simulink model "SpinningMode"  (R2024b)
settings: Solver=FixedStepAuto  StartTime=0.0  StopTime=10.0  RelTol=1e-3  EnableMultiTasking=on
undefined symbols (not defined in the file): MSpin, nRPMSpinningModeIntegralActivation, NSpinningModeKi, NSpinningModelKp, nTargetRPM, tSpinLength, tTorqueControlTask
libraries: simulink x3, simulink_extras x1
settings Model: DataDictionary=Master_Dictionary.sldd  EnableAccessToBaseWorkspace=off  Creator=torni  LastModifiedBy=Will
settings OptimizationCC: DefaultParameterBehavior=Inlined  EnhancedBackFolding=on  PassReuseOutputArgsAs=Individual arguments  ZeroExternalMemoryAtStartup=off  ZeroInternalMemoryAtStartup=off  MaxStackSize=8192  OptimizeBlockOrder=speed  DifferentSizesBufferReuse=on  OptimizationCustomize=off  EfficientTunableParamExpr=on
settings DebuggingCC: ParameterTunabilityLossMsg=error
settings HardwareCC: ProdBitPerPointer=32  ProdBitPerSizeT=32  ProdBitPerPtrDiffT=32  ProdLargestAtomicInteger=Long  ProdLargestAtomicFloat=Double  ProdWordSize=32  ProdLongLongMode=on  ProdHWDeviceType=ARM Compatible->ARM Cortex-M
settings SFSimCC: MATLABDynamicMemAlloc=off
settings RTWCC: Description=Embedded Coder  SystemTargetFile=ert.tlc  HardwareBoard=STM32H7xx Based (Single-core)  TemplateMakefile=ert_default_tmf  Toolchain=GNU Tools for ARM Embedded Processors
settings CodeAppCC: ForceParamTrailComments=on  IgnoreCustomStorageClasses=off  OperatorAnnotations=on  SimulinkDataObjDesc=on  SFDataObjDesc=on  InsertBlockDesc=on
settings ERTTargetCC: TargetLangStandard=C99 (ISO)  CodeReplacementLibrary=ARM Cortex-M  ExtModeTransport=3  ExtModeStaticAlloc=on  ExtModeStaticAllocSize=2048  ExtModeMexFile=ext_xcp  ExtModeIntrfLevel=Level2 - Open

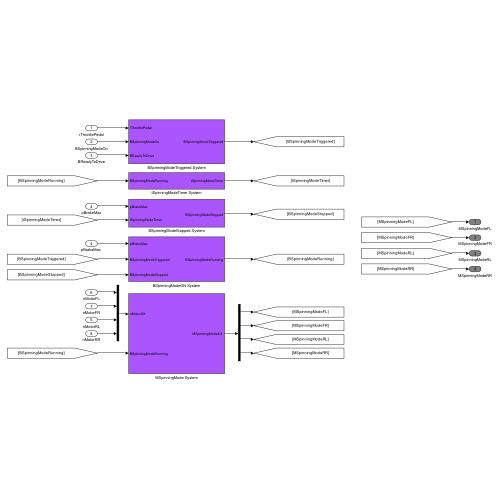
[thumbnail: Simulink's stored preview of the top-level diagram]
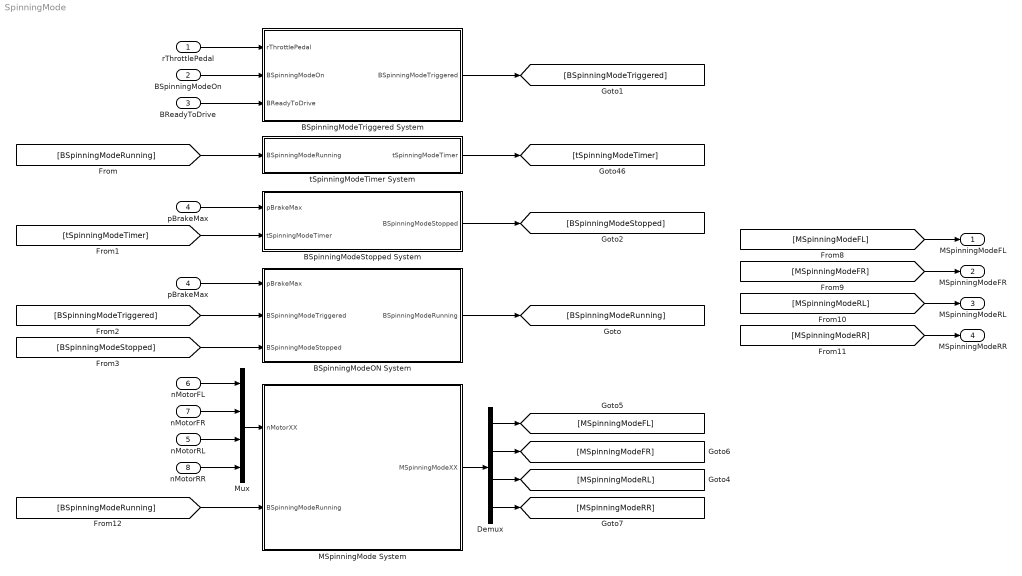
== system SpinningMode ==
  rThrottlePedal : Inport  OutDataTypeStr=double
  "BSpinningModeOn " : Inport  Port=2  OutDataTypeStr=boolean
  BReadyToDrive : Inport  Port=3  OutDataTypeStr=boolean
  pBrakeMax : Inport  Port=4  OutDataTypeStr=double
  nMotorRL : Inport  Port=5  OutDataTypeStr=double
  nMotorFL : Inport  Port=6  OutDataTypeStr=double
  nMotorFR : Inport  Port=7  OutDataTypeStr=double
  nMotorRR : Inport  Port=8  OutDataTypeStr=double
  BSpinningModeON System : Subsystem
  BSpinningModeStopped System : Subsystem
  BSpinningModeTriggered System : Subsystem
  Demux : Demux
  MSpinningMode System : Subsystem
  Mux : Mux
  "pBrakeMax " : InportShadow  Port=4  OutDataTypeStr=double
  tSpinningModeTimer System : Subsystem
  MSpinningModeFL : Outport  OutDataTypeStr=double  VectorParamsAs1DForOutWhenUnconnected=off
  MSpinningModeFR : Outport  Port=2  OutDataTypeStr=double  VectorParamsAs1DForOutWhenUnconnected=off
  MSpinningModeRL : Outport  Port=3  OutDataTypeStr=double  VectorParamsAs1DForOutWhenUnconnected=off
  MSpinningModeRR : Outport  Port=4  OutDataTypeStr=double  VectorParamsAs1DForOutWhenUnconnected=off
  wires:
  rThrottlePedal/1 -> BSpinningModeTriggered System/1(rThrottlePedal)
  "BSpinningModeOn "/1 -> BSpinningModeTriggered System/2("BSpinningModeOn ")
  BReadyToDrive/1 -> BSpinningModeTriggered System/3(BReadyToDrive)
  pBrakeMax/1 -> BSpinningModeStopped System/1(pBrakeMax)
  [tSpinningModeTimer] -> BSpinningModeStopped System/2(tSpinningModeTimer)
  tSpinningModeTimer System/1(tSpinningModeTimer) -> [tSpinningModeTimer]
  BSpinningModeTriggered System/1(BSpinningModeTriggered) -> [BSpinningModeTriggered]
  BSpinningModeStopped System/1(BSpinningModeStopped) -> [BSpinningModeStopped]
  "pBrakeMax "/1 -> BSpinningModeON System/1(pBrakeMax)
  [BSpinningModeTriggered] -> BSpinningModeON System/2(BSpinningModeTriggered)
  [BSpinningModeStopped] -> BSpinningModeON System/3(BSpinningModeStopped)
  BSpinningModeON System/1(BSpinningModeRunning) -> [BSpinningModeRunning]
  [BSpinningModeRunning] -> tSpinningModeTimer System/1(BSpinningModeRunning)
  Demux/3 -> [MSpinningModeRL]
  Demux/1 -> [MSpinningModeFL]
  Demux/2 -> [MSpinningModeFR]
  Demux/4 -> [MSpinningModeRR]
  [MSpinningModeFL] -> MSpinningModeFL/1
  [MSpinningModeFR] -> MSpinningModeFR/1
  [MSpinningModeRR] -> MSpinningModeRR/1
  [MSpinningModeRL] -> MSpinningModeRL/1
  Mux/1 -> MSpinningMode System/1(nMotorXX)
  nMotorFL/1 -> Mux/1
  nMotorFR/1 -> Mux/2
  nMotorRL/1 -> Mux/3
  nMotorRR/1 -> Mux/4
  [BSpinningModeRunning] -> MSpinningMode System/2(BSpinningModeRunning)
  MSpinningMode System/1("MSpinningModeXX ") -> Demux/1

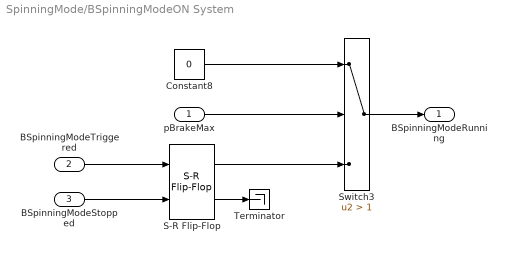
== system SpinningMode/BSpinningModeON System ==
  pBrakeMax : Inport  OutDataTypeStr=double
  BSpinningModeTriggered : Inport  Port=2  OutDataTypeStr=boolean
  BSpinningModeStopped : Inport  Port=3  OutDataTypeStr=boolean
  Constant8 : Constant  Value=0
  S-R Flip-Flop : simulink_extras/Flip Flops/S-R Flip-Flop  initial_condition=0
  Switch3 : Switch  Criteria=u2 > Threshold  Threshold=1  SaturateOnIntegerOverflow=off  InputSameDT=off
  Terminator : Terminator
  BSpinningModeRunning : Outport  OutDataTypeStr=boolean  VectorParamsAs1DForOutWhenUnconnected=off
  wires:
  Switch3/1 -> BSpinningModeRunning/1
  BSpinningModeTriggered/1 -> S-R Flip-Flop/1
  Constant8/1 -> Switch3/1
  S-R Flip-Flop/1 -> Switch3/3
  S-R Flip-Flop/2 -> Terminator/1
  BSpinningModeStopped/1 -> S-R Flip-Flop/2
  pBrakeMax/1 -> Switch3/2

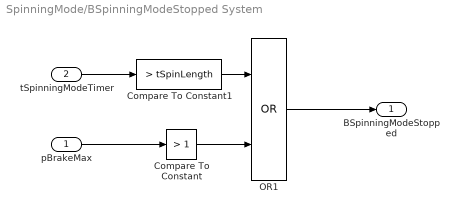
== system SpinningMode/BSpinningModeStopped System ==
  pBrakeMax : Inport  OutDataTypeStr=double
  tSpinningModeTimer : Inport  Port=2  OutDataTypeStr=double
  Compare To Constant : simulink/Logic and Bit Operations/Compare To Constant  relop=>  const=1  OutDataTypeStr=boolean
  Compare To Constant1 : simulink/Logic and Bit Operations/Compare To Constant  relop=>  const=tSpinLength  OutDataTypeStr=boolean
  OR1 : Logic  Operator=OR  AllPortsSameDT=off  OutDataTypeStr=boolean
  BSpinningModeStopped : Outport  OutDataTypeStr=boolean  VectorParamsAs1DForOutWhenUnconnected=off
  wires:
  Compare To Constant1/1 -> OR1/1
  Compare To Constant/1 -> OR1/2
  OR1/1 -> BSpinningModeStopped/1
  pBrakeMax/1 -> Compare To Constant/1
  tSpinningModeTimer/1 -> Compare To Constant1/1

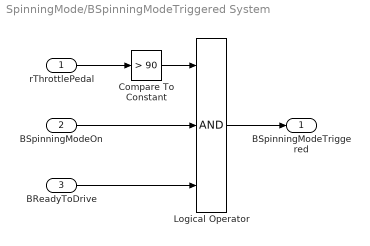
== system SpinningMode/BSpinningModeTriggered System ==
  rThrottlePedal : Inport  OutDataTypeStr=double
  "BSpinningModeOn " : Inport  Port=2  OutDataTypeStr=boolean
  BReadyToDrive : Inport  Port=3  OutDataTypeStr=boolean
  Compare To Constant : simulink/Logic and Bit Operations/Compare To Constant  relop=>  const=90  OutDataTypeStr=boolean
  Logical Operator : Logic  Inputs=3  AllPortsSameDT=off  OutDataTypeStr=boolean
  BSpinningModeTriggered : Outport  OutDataTypeStr=boolean  VectorParamsAs1DForOutWhenUnconnected=off
  wires:
  Logical Operator/1 -> BSpinningModeTriggered/1
  "BSpinningModeOn "/1 -> Logical Operator/2
  rThrottlePedal/1 -> Compare To Constant/1
  Compare To Constant/1 -> Logical Operator/1
  BReadyToDrive/1 -> Logical Operator/3

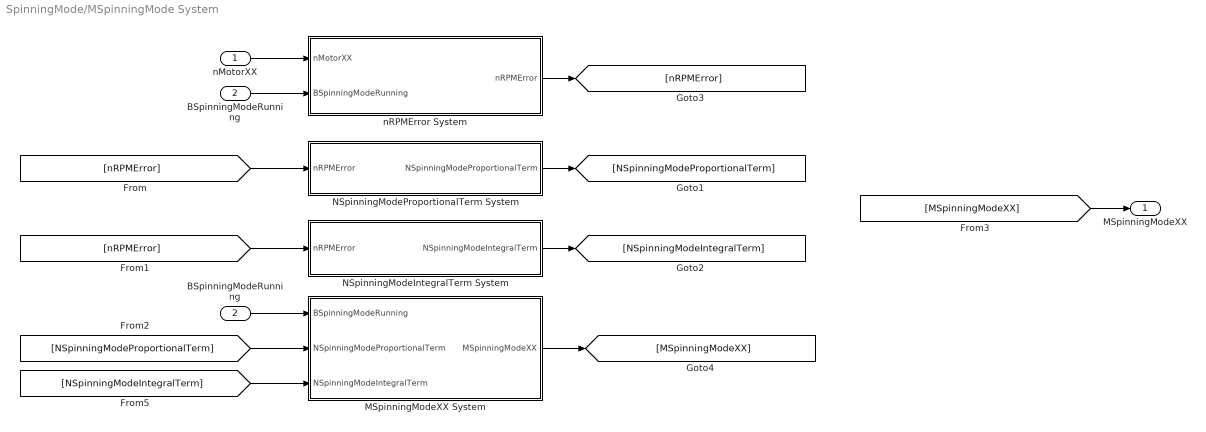
== system SpinningMode/MSpinningMode System ==
  nMotorXX : Inport  OutDataTypeStr=double
  BSpinningModeRunning : Inport  Port=2  OutDataTypeStr=boolean
  "BSpinningModeRunning " : InportShadow  Port=2  OutDataTypeStr=boolean
  MSpinningModeXX System : Subsystem
  NSpinningModeIntegralTerm System : Subsystem
  NSpinningModeProportionalTerm System : Subsystem
  nRPMError System : Subsystem
  "MSpinningModeXX " : Outport  OutDataTypeStr=double  VectorParamsAs1DForOutWhenUnconnected=off
  wires:
  nMotorXX/1 -> nRPMError System/1(nMotorXX)
  BSpinningModeRunning/1 -> nRPMError System/2(BSpinningModeRunning)
  nRPMError System/1(nRPMError) -> [nRPMError]
  [nRPMError] -> NSpinningModeProportionalTerm System/1(nRPMError)
  NSpinningModeProportionalTerm System/1(NSpinningModeProportionalTerm) -> [NSpinningModeProportionalTerm]
  [nRPMError] -> NSpinningModeIntegralTerm System/1(nRPMError)
  NSpinningModeIntegralTerm System/1("NSpinningModeIntegralTerm ") -> [NSpinningModeIntegralTerm]
  [NSpinningModeProportionalTerm] -> MSpinningModeXX System/2(NSpinningModeProportionalTerm)
  [NSpinningModeIntegralTerm] -> MSpinningModeXX System/3(NSpinningModeIntegralTerm)
  "BSpinningModeRunning "/1 -> MSpinningModeXX System/1(BSpinningModeRunning)
  MSpinningModeXX System/1("MSpinningModeXX ") -> [MSpinningModeXX]
  [MSpinningModeXX] -> "MSpinningModeXX "/1

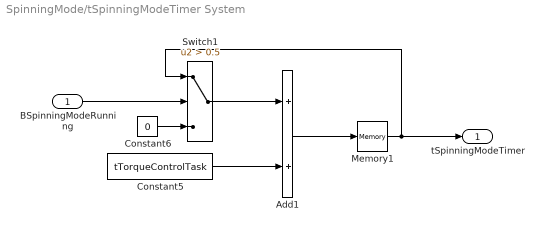
== system SpinningMode/tSpinningModeTimer System ==
  BSpinningModeRunning : Inport  OutDataTypeStr=boolean
  Add1 : Sum
  Constant5 : Constant  Value=tTorqueControlTask
  Constant6 : Constant  Value=0
  Memory1 : Memory  InheritSampleTime=on
  Switch1 : Switch  Criteria=u2 > Threshold  Threshold=0.5  SaturateOnIntegerOverflow=off  InputSameDT=off
  tSpinningModeTimer : Outport  OutDataTypeStr=double  VectorParamsAs1DForOutWhenUnconnected=off
  wires:
  Add1/1 -> Memory1/1
  Memory1/1 -> tSpinningModeTimer/1, Switch1/1
  Switch1/1 -> Add1/1
  Constant5/1 -> Add1/2
  Constant6/1 -> Switch1/3
  BSpinningModeRunning/1 -> Switch1/2

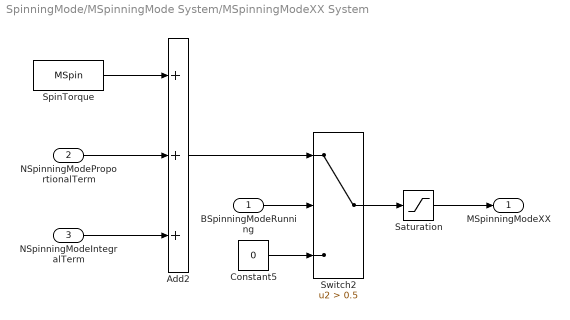
== system SpinningMode/MSpinningMode System/MSpinningModeXX System ==
  BSpinningModeRunning : Inport  OutDataTypeStr=boolean
  NSpinningModeProportionalTerm : Inport  Port=2  OutDataTypeStr=double
  NSpinningModeIntegralTerm : Inport  Port=3  OutDataTypeStr=double
  Add2 : Sum  Inputs=+++
  Constant5 : Constant  Value=0
  Saturation : Saturate  UpperLimit=15  LowerLimit=0
  SpinTorque : Constant  Value=MSpin
  Switch2 : Switch  Criteria=u2 > Threshold  Threshold=0.5  SaturateOnIntegerOverflow=off  InputSameDT=off
  "MSpinningModeXX " : Outport  OutDataTypeStr=double  VectorParamsAs1DForOutWhenUnconnected=off
  wires:
  Switch2/1 -> Saturation/1
  SpinTorque/1 -> Add2/1
  Constant5/1 -> Switch2/3
  BSpinningModeRunning/1 -> Switch2/2
  Add2/1 -> Switch2/1
  Saturation/1 -> "MSpinningModeXX "/1
  NSpinningModeProportionalTerm/1 -> Add2/2
  NSpinningModeIntegralTerm/1 -> Add2/3

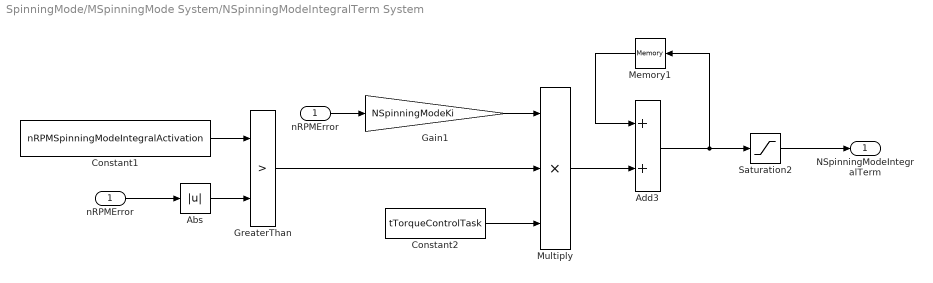
== system SpinningMode/MSpinningMode System/NSpinningModeIntegralTerm System ==
  nRPMError : Inport  OutDataTypeStr=double
  Abs : Abs  SaturateOnIntegerOverflow=off
  Add3 : Sum
  Constant1 : Constant  Value=nRPMSpinningModeIntegralActivation  VectorParams1D=off
  Constant2 : Constant  Value=tTorqueControlTask
  Gain1 : Gain  Gain=NSpinningModeKi
  GreaterThan : RelationalOperator  Operator=>  OutDataTypeStr=boolean  RndMeth=Simplest  InputSameDT=off
  Memory1 : Memory  InheritSampleTime=on
  Multiply : Product  Inputs=3
  Saturation2 : Saturate  UpperLimit=3  LowerLimit=-3
  "nRPMError " : InportShadow  OutDataTypeStr=double
  "NSpinningModeIntegralTerm " : Outport  OutDataTypeStr=double  VectorParamsAs1DForOutWhenUnconnected=off
  wires:
  Memory1/1 -> Add3/1
  Gain1/1 -> Multiply/1
  Add3/1 -> Saturation2/1, Memory1/1
  Constant1/1 -> GreaterThan/1
  Multiply/1 -> Add3/2
  "nRPMError "/1 -> Gain1/1
  Abs/1 -> GreaterThan/2
  GreaterThan/1 -> Multiply/2
  nRPMError/1 -> Abs/1
  Constant2/1 -> Multiply/3
  Saturation2/1 -> "NSpinningModeIntegralTerm "/1

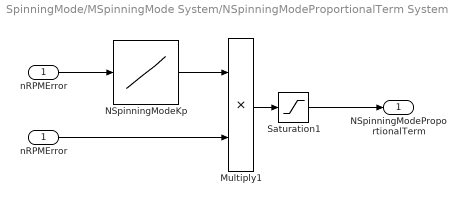
== system SpinningMode/MSpinningMode System/NSpinningModeProportionalTerm System ==
  nRPMError : Inport  OutDataTypeStr=double
  Multiply1 : Product
  NSpinningModeKp : Lookup_n-D  NumberOfTableDimensions=1  BreakpointsForDimension1=[-3000, 0, 3000]  BreakpointsForDimension2=[1:3]  Table=[NSpinningModelKp, 0, NSpinningModelKp]  InternalRulePriority=Speed  RndMeth=Simplest
  Saturation1 : Saturate  UpperLimit=7  LowerLimit=-7
  "nRPMError " : InportShadow  OutDataTypeStr=double
  NSpinningModeProportionalTerm : Outport  OutDataTypeStr=double  VectorParamsAs1DForOutWhenUnconnected=off
  wires:
  nRPMError/1 -> NSpinningModeKp/1
  NSpinningModeKp/1 -> Multiply1/1
  Multiply1/1 -> Saturation1/1
  "nRPMError "/1 -> Multiply1/2
  Saturation1/1 -> NSpinningModeProportionalTerm/1

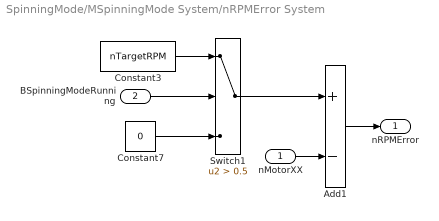
== system SpinningMode/MSpinningMode System/nRPMError System ==
  nMotorXX : Inport  OutDataTypeStr=double
  BSpinningModeRunning : Inport  Port=2  OutDataTypeStr=boolean
  Add1 : Sum  Inputs=+-
  Constant3 : Constant  Value=nTargetRPM
  Constant7 : Constant  Value=0
  Switch1 : Switch  Criteria=u2 > Threshold  Threshold=0.5  SaturateOnIntegerOverflow=off  InputSameDT=off
  nRPMError : Outport  OutDataTypeStr=double  VectorParamsAs1DForOutWhenUnconnected=off
  wires:
  BSpinningModeRunning/1 -> Switch1/2
  Add1/1 -> nRPMError/1
  Constant3/1 -> Switch1/1
  Constant7/1 -> Switch1/3
  nMotorXX/1 -> Add1/2
  Switch1/1 -> Add1/1
